simulink subsystem "SubSystemHubmagnetVereinzelung"  (R2020b)
settings: Solver=VariableStepAuto  StartTime=0.0  StopTime=10.0  RelTol=1e-3
settings Model: Creator=kaebi  LastModifiedBy=kaebi

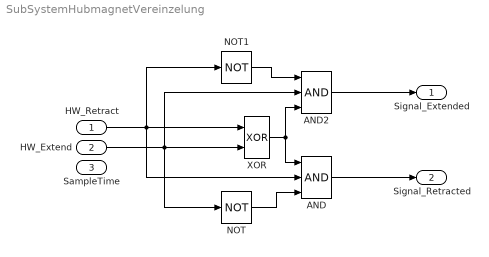
== system SubSystemHubmagnetVereinzelung ==
  HW_Retract : Inport
  HW_Extend : Inport  Port=2
  SampleTime : Inport  Port=3
  AND : Logic  Inputs=3  IconShape=distinctive  AllPortsSameDT=off  OutDataTypeStr=boolean
  AND2 : Logic  Inputs=3  IconShape=distinctive  AllPortsSameDT=off  OutDataTypeStr=boolean
  NOT : Logic  Operator=NOT  IconShape=distinctive  AllPortsSameDT=off  OutDataTypeStr=boolean
  NOT1 : Logic  Operator=NOT  IconShape=distinctive  AllPortsSameDT=off  OutDataTypeStr=boolean
  XOR : Logic  Operator=XOR  IconShape=distinctive  AllPortsSameDT=off  OutDataTypeStr=boolean
  Signal_Extended : Outport
  Signal_Retracted : Outport  Port=2
  wires:
  NOT/1 -> AND/3
  HW_Retract/1 -> AND/2, NOT1/1, XOR/1
  HW_Extend/1 -> XOR/2, AND2/2, NOT/1
  AND/1 -> Signal_Retracted/1
  AND2/1 -> Signal_Extended/1
  NOT1/1 -> AND2/1
  XOR/1 -> AND/1, AND2/3
